simulink model "Shanthan_Heeirthan_EE469S3D_R45 (1)"  (R2023a)
settings: Solver=FixedStepDiscrete  StartTime=0.0  StopTime=120  FixedStep=dt0  RelTol=1e-3  EnableMultiTasking=on
PostLoadFcn:
  | %Set the size for the model
  | set_param(gcs,'Location',[10 10 1270 970])
  | %Set the zoom factor for the model
  | set_param(gcs,'ZoomFactor','100')
InitFcn:
  | tic
  | % Students Add call to their M-file HERE
  | Shanthan_Heeirthan_EE460_Final
  | INIT_S3D_01
StartFcn:
  | tend0=toc;
  | tic;
StopFcn:
  | tend=toc;
  | disp(['Simulation time = ' num2str(tout(end)) ' sec'])
  | disp(['Real time = ' num2str(tend) ' sec'])
  | title('DONE')
  | SCORE=round((max(0,120-tout(end)-tend0))*4+10*(40-FuelBurned)+sum(100*double(PDONE)-100*double(PDONE<.5)));
  | PlotS3D(PlotInput);
  | text(15,22,['S: ' num2str(SCORE)]);
values from neighbouring files (symbols this model uses):
  A = [0 1 0 0 0 0 ... (first row only)    [Shanthan_Heeirthan_EE460_Final (1).m]
  B = [0 0 0 ... (first row only)    [Shanthan_Heeirthan_EE460_Final (1).m]
  bm = [1 1 -1 -1 0 0 0 0; 0 0 0 0 -1 1 1 -1; -1 1 -1 1 3 -3 3 -3]    [Shanthan_Heeirthan_EE460_Final (1).m]
  C = [1 0 0 0 0 0 ... (first row only)    [Shanthan_Heeirthan_EE460_Final (1).m]
  D = [0 0 0 ... (first row only)    [Shanthan_Heeirthan_EE460_Final (1).m]
  Denchptheta = TFchptheta.Den{1}    [Shanthan_Heeirthan_EE460_Final (1).m]
  Denchpxy = TFchpxy.Den{1}    [Shanthan_Heeirthan_EE460_Final (1).m]
  Denclptheta = TFclptheta.Den{1}    [Shanthan_Heeirthan_EE460_Final (1).m]
  Denclpxy = TFclpxy.Den{1}    [Shanthan_Heeirthan_EE460_Final (1).m]
  Denlp = TFlp.Den{1}    [Shanthan_Heeirthan_EE460_Final (1).m]
  Kd = 2.1+0    (= 2.1)    [Shanthan_Heeirthan_EE460_Final (1).m]
  Ki = 0.0001    [Shanthan_Heeirthan_EE460_Final (1).m]
  Kp = 1.1+0.2    (= 1.3)    [Shanthan_Heeirthan_EE460_Final (1).m]
  L = place(A',C',ep)'    [Shanthan_Heeirthan_EE460_Final (1).m]
  Numchptheta = TFchptheta.Num{1}    [Shanthan_Heeirthan_EE460_Final (1).m]
  Numchpxy = TFchpxy.Num{1}    [Shanthan_Heeirthan_EE460_Final (1).m]
  Numclptheta = TFclptheta.Num{1}    [Shanthan_Heeirthan_EE460_Final (1).m]
  Numclpxy = TFclpxy.Num{1}    [Shanthan_Heeirthan_EE460_Final (1).m]
  Numlp = TFlp.Num{1}    [Shanthan_Heeirthan_EE460_Final (1).m]
  Pnewdata = [LVL.P1 LVL.P2 LVL.P3 LVL.P4]    [Shanthan_Heeirthan_EE460_Final (1).m]
  Sconfig = 1    [Shanthan_Heeirthan_EE460_Final (1).m]
  TFP1 = 2    [Shanthan_Heeirthan_EE460_Final (1).m]
  TFP1z = 1    [Shanthan_Heeirthan_EE460_Final (1).m]
  TFP2 = 2    [Shanthan_Heeirthan_EE460_Final (1).m]
  TFP2z = 1    [Shanthan_Heeirthan_EE460_Final (1).m]
  TFP3 = 2    [Shanthan_Heeirthan_EE460_Final (1).m]
  TFP3z = 1    [Shanthan_Heeirthan_EE460_Final (1).m]
  TFP4 = 2    [Shanthan_Heeirthan_EE460_Final (1).m]
  TFP4z = 1    [Shanthan_Heeirthan_EE460_Final (1).m]
  wcf = 2    [Shanthan_Heeirthan_EE460_Final (1).m]
  wcft = 10    [Shanthan_Heeirthan_EE460_Final (1).m]
undefined symbols (not defined in the file or in its folder): d2r, DiscIntNeverNeededParam, dt, dt0, fr, HM_S, HM_U, J, Jbase, JC0, L13, L24, LVL, M, M1, M2, M3, M4, mdti, Pdata, PTvec, r2d, SLIM, SQ, SSF, TOLdata, ULIM
libraries: simulink x85, aerolibanimutils x1, matrix_library x1
(part 5 of 7)

== system Shanthan_Heeirthan_EE469S3D_R45 (1)/S3D_Plant/Sensors/CASE1/Xaccel/CURRENT ==
  In1 : Inport
  Action Port : ActionPort  ActionPortLabel=else
  Out1 : Outport
  wires:
  In1/1 -> Out1/1

== system Shanthan_Heeirthan_EE469S3D_R45 (1)/S3D_Plant/Sensors/CASE1/Xaccel/MAX ==
  Action Port : ActionPort  ActionPortLabel=elseif(u1 > 0.5 & u1 < 1.5)
  Constant : Constant  Value=SLIM(3,2)  SampleTime=dt0
  Out1 : Outport
  wires:
  Constant/1 -> Out1/1

== system Shanthan_Heeirthan_EE469S3D_R45 (1)/S3D_Plant/Sensors/CASE1/Xaccel/MIN ==
  Action Port : ActionPort  ActionPortLabel=if(u1 < -0.5)
  Constant : Constant  Value=SLIM(3,1)  SampleTime=dt0
  Out1 : Outport
  wires:
  Constant/1 -> Out1/1

== system Shanthan_Heeirthan_EE469S3D_R45 (1)/S3D_Plant/Sensors/CASE1/Xpos1/CURRENT ==
  In1 : Inport
  Action Port : ActionPort  ActionPortLabel=else
  Out1 : Outport
  wires:
  In1/1 -> Out1/1

== system Shanthan_Heeirthan_EE469S3D_R45 (1)/S3D_Plant/Sensors/CASE1/Xpos1/MAX ==
  Action Port : ActionPort  ActionPortLabel=elseif(u1 > 0.5 & u1 < 1.5)
  Constant : Constant  Value=SLIM(1,2)  SampleTime=dt0
  Out1 : Outport
  wires:
  Constant/1 -> Out1/1

== system Shanthan_Heeirthan_EE469S3D_R45 (1)/S3D_Plant/Sensors/CASE1/Xpos1/MIN ==
  Action Port : ActionPort  ActionPortLabel=if(u1 < -0.5)
  Constant : Constant  Value=SLIM(1,1)  SampleTime=dt0
  Out1 : Outport
  wires:
  Constant/1 -> Out1/1

== system Shanthan_Heeirthan_EE469S3D_R45 (1)/S3D_Plant/Sensors/CASE1/Xvel/CURRENT ==
  In1 : Inport
  Action Port : ActionPort  ActionPortLabel=else
  Out1 : Outport
  wires:
  In1/1 -> Out1/1

== system Shanthan_Heeirthan_EE469S3D_R45 (1)/S3D_Plant/Sensors/CASE1/Xvel/MAX ==
  Action Port : ActionPort  ActionPortLabel=elseif(u1 > 0.5 & u1 < 1.5)
  Constant : Constant  Value=SLIM(2,2)  SampleTime=dt0
  Out1 : Outport
  wires:
  Constant/1 -> Out1/1

== system Shanthan_Heeirthan_EE469S3D_R45 (1)/S3D_Plant/Sensors/CASE1/Xvel/MIN ==
  Action Port : ActionPort  ActionPortLabel=if(u1 < -0.5)
  Constant : Constant  Value=SLIM(2,1)  SampleTime=dt0
  Out1 : Outport
  wires:
  Constant/1 -> Out1/1

== system Shanthan_Heeirthan_EE469S3D_R45 (1)/S3D_Plant/Sensors/CASE1/Yaccel/CURRENT ==
  In1 : Inport
  Action Port : ActionPort  ActionPortLabel=else
  Out1 : Outport
  wires:
  In1/1 -> Out1/1

== system Shanthan_Heeirthan_EE469S3D_R45 (1)/S3D_Plant/Sensors/CASE1/Yaccel/MAX ==
  Action Port : ActionPort  ActionPortLabel=elseif(u1 > 0.5 & u1 < 1.5)
  Constant : Constant  Value=SLIM(6,2)  SampleTime=dt0
  Out1 : Outport
  wires:
  Constant/1 -> Out1/1

== system Shanthan_Heeirthan_EE469S3D_R45 (1)/S3D_Plant/Sensors/CASE1/Yaccel/MIN ==
  Action Port : ActionPort  ActionPortLabel=if(u1 < -0.5)
  Constant : Constant  Value=SLIM(6,1)  SampleTime=dt0
  Out1 : Outport
  wires:
  Constant/1 -> Out1/1

== system Shanthan_Heeirthan_EE469S3D_R45 (1)/S3D_Plant/Sensors/CASE1/Ypos1/CURRENT ==
  In1 : Inport
  Action Port : ActionPort  ActionPortLabel=else
  Out1 : Outport
  wires:
  In1/1 -> Out1/1

== system Shanthan_Heeirthan_EE469S3D_R45 (1)/S3D_Plant/Sensors/CASE1/Ypos1/MAX ==
  Action Port : ActionPort  ActionPortLabel=elseif(u1 > 0.5 & u1 < 1.5)
  Constant : Constant  Value=SLIM(4,2)  SampleTime=dt0
  Out1 : Outport
  wires:
  Constant/1 -> Out1/1

== system Shanthan_Heeirthan_EE469S3D_R45 (1)/S3D_Plant/Sensors/CASE1/Ypos1/MIN ==
  Action Port : ActionPort  ActionPortLabel=if(u1 < -0.5)
  Constant : Constant  Value=SLIM(4,1)  SampleTime=dt0
  Out1 : Outport
  wires:
  Constant/1 -> Out1/1

== system Shanthan_Heeirthan_EE469S3D_R45 (1)/S3D_Plant/Sensors/CASE1/Yvel/CURRENT ==
  In1 : Inport
  Action Port : ActionPort  ActionPortLabel=else
  Out1 : Outport
  wires:
  In1/1 -> Out1/1

== system Shanthan_Heeirthan_EE469S3D_R45 (1)/S3D_Plant/Sensors/CASE1/Yvel/MAX ==
  Action Port : ActionPort  ActionPortLabel=elseif(u1 > 0.5 & u1 < 1.5)
  Constant : Constant  Value=SLIM(5,2)  SampleTime=dt0
  Out1 : Outport
  wires:
  Constant/1 -> Out1/1

== system Shanthan_Heeirthan_EE469S3D_R45 (1)/S3D_Plant/Sensors/CASE1/Yvel/MIN ==
  Action Port : ActionPort  ActionPortLabel=if(u1 < -0.5)
  Constant : Constant  Value=SLIM(5,1)  SampleTime=dt0
  Out1 : Outport
  wires:
  Constant/1 -> Out1/1

== system Shanthan_Heeirthan_EE469S3D_R45 (1)/S3D_Plant/Sensors/CASE2/THTpos1/CURRENT ==
  In1 : Inport
  Action Port : ActionPort  ActionPortLabel=else
  Out1 : Outport
  wires:
  In1/1 -> Out1/1

== system Shanthan_Heeirthan_EE469S3D_R45 (1)/S3D_Plant/Sensors/CASE2/THTpos1/MAX ==
  Action Port : ActionPort  ActionPortLabel=elseif(u1 > 0.5 & u1 < 1.5)
  Constant : Constant  Value=SLIM(7,2)  SampleTime=dt0
  Out1 : Outport
  wires:
  Constant/1 -> Out1/1

== system Shanthan_Heeirthan_EE469S3D_R45 (1)/S3D_Plant/Sensors/CASE2/THTpos1/MIN ==
  Action Port : ActionPort  ActionPortLabel=if(u1 < -0.5)
  Constant : Constant  Value=SLIM(7,1)  SampleTime=dt0
  Out1 : Outport
  wires:
  Constant/1 -> Out1/1

== system Shanthan_Heeirthan_EE469S3D_R45 (1)/S3D_Plant/Sensors/CASE2/THTpos2/CURRENT ==
  In1 : Inport
  Action Port : ActionPort  ActionPortLabel=else
  Out1 : Outport
  wires:
  In1/1 -> Out1/1

== system Shanthan_Heeirthan_EE469S3D_R45 (1)/S3D_Plant/Sensors/CASE2/THTpos2/MAX ==
  Action Port : ActionPort  ActionPortLabel=elseif(u1 > 0.5 & u1 < 1.5)
  Constant : Constant  Value=SLIM(7,2)  SampleTime=dt0
  Out1 : Outport
  wires:
  Constant/1 -> Out1/1

== system Shanthan_Heeirthan_EE469S3D_R45 (1)/S3D_Plant/Sensors/CASE2/THTpos2/MIN ==
  Action Port : ActionPort  ActionPortLabel=if(u1 < -0.5)
  Constant : Constant  Value=SLIM(7,1)  SampleTime=dt0
  Out1 : Outport
  wires:
  Constant/1 -> Out1/1

== system Shanthan_Heeirthan_EE469S3D_R45 (1)/S3D_Plant/Sensors/CASE2/THTvel/CURRENT ==
  In1 : Inport
  Action Port : ActionPort  ActionPortLabel=else
  Out1 : Outport
  wires:
  In1/1 -> Out1/1

== system Shanthan_Heeirthan_EE469S3D_R45 (1)/S3D_Plant/Sensors/CASE2/THTvel/MAX ==
  Action Port : ActionPort  ActionPortLabel=elseif(u1 > 0.5 & u1 < 1.5)
  Constant : Constant  Value=SLIM(8,2)  SampleTime=dt0
  Out1 : Outport
  wires:
  Constant/1 -> Out1/1

== system Shanthan_Heeirthan_EE469S3D_R45 (1)/S3D_Plant/Sensors/CASE2/THTvel/MIN ==
  Action Port : ActionPort  ActionPortLabel=if(u1 < -0.5)
  Constant : Constant  Value=SLIM(8,1)  SampleTime=dt0
  Out1 : Outport
  wires:
  Constant/1 -> Out1/1

== system Shanthan_Heeirthan_EE469S3D_R45 (1)/S3D_Plant/Sensors/CASE2/Xpos1/CURRENT ==
  In1 : Inport
  Action Port : ActionPort  ActionPortLabel=else
  Out1 : Outport
  wires:
  In1/1 -> Out1/1

== system Shanthan_Heeirthan_EE469S3D_R45 (1)/S3D_Plant/Sensors/CASE2/Xpos1/MAX ==
  Action Port : ActionPort  ActionPortLabel=elseif(u1 > 0.5 & u1 < 1.5)
  Constant : Constant  Value=SLIM(1,2)  SampleTime=dt0
  Out1 : Outport
  wires:
  Constant/1 -> Out1/1

== system Shanthan_Heeirthan_EE469S3D_R45 (1)/S3D_Plant/Sensors/CASE2/Xpos1/MIN ==
  Action Port : ActionPort  ActionPortLabel=if(u1 < -0.5)
  Constant : Constant  Value=SLIM(1,1)  SampleTime=dt0
  Out1 : Outport
  wires:
  Constant/1 -> Out1/1

== system Shanthan_Heeirthan_EE469S3D_R45 (1)/S3D_Plant/Sensors/CASE2/Xpos2/CURRENT ==
  In1 : Inport
  Action Port : ActionPort  ActionPortLabel=else
  Out1 : Outport
  wires:
  In1/1 -> Out1/1

== system Shanthan_Heeirthan_EE469S3D_R45 (1)/S3D_Plant/Sensors/CASE2/Xpos2/MAX ==
  Action Port : ActionPort  ActionPortLabel=elseif(u1 > 0.5 & u1 < 1.5)
  Constant : Constant  Value=SLIM(1,2)  SampleTime=dt0
  Out1 : Outport
  wires:
  Constant/1 -> Out1/1

== system Shanthan_Heeirthan_EE469S3D_R45 (1)/S3D_Plant/Sensors/CASE2/Xpos2/MIN ==
  Action Port : ActionPort  ActionPortLabel=if(u1 < -0.5)
  Constant : Constant  Value=SLIM(1,1)  SampleTime=dt0
  Out1 : Outport
  wires:
  Constant/1 -> Out1/1

== system Shanthan_Heeirthan_EE469S3D_R45 (1)/S3D_Plant/Sensors/CASE2/Xvel/CURRENT ==
  In1 : Inport
  Action Port : ActionPort  ActionPortLabel=else
  Out1 : Outport
  wires:
  In1/1 -> Out1/1

== system Shanthan_Heeirthan_EE469S3D_R45 (1)/S3D_Plant/Sensors/CASE2/Xvel/MAX ==
  Action Port : ActionPort  ActionPortLabel=elseif(u1 > 0.5 & u1 < 1.5)
  Constant : Constant  Value=SLIM(2,2)  SampleTime=dt0
  Out1 : Outport
  wires:
  Constant/1 -> Out1/1

== system Shanthan_Heeirthan_EE469S3D_R45 (1)/S3D_Plant/Sensors/CASE2/Xvel/MIN ==
  Action Port : ActionPort  ActionPortLabel=if(u1 < -0.5)
  Constant : Constant  Value=SLIM(2,1)  SampleTime=dt0
  Out1 : Outport
  wires:
  Constant/1 -> Out1/1

== system Shanthan_Heeirthan_EE469S3D_R45 (1)/S3D_Plant/Sensors/CASE2/Ypos1/CURRENT ==
  In1 : Inport
  Action Port : ActionPort  ActionPortLabel=else
  Out1 : Outport
  wires:
  In1/1 -> Out1/1

== system Shanthan_Heeirthan_EE469S3D_R45 (1)/S3D_Plant/Sensors/CASE2/Ypos1/MAX ==
  Action Port : ActionPort  ActionPortLabel=elseif(u1 > 0.5 & u1 < 1.5)
  Constant : Constant  Value=SLIM(4,2)  SampleTime=dt0
  Out1 : Outport
  wires:
  Constant/1 -> Out1/1

== system Shanthan_Heeirthan_EE469S3D_R45 (1)/S3D_Plant/Sensors/CASE2/Ypos1/MIN ==
  Action Port : ActionPort  ActionPortLabel=if(u1 < -0.5)
  Constant : Constant  Value=SLIM(4,1)  SampleTime=dt0
  Out1 : Outport
  wires:
  Constant/1 -> Out1/1

== system Shanthan_Heeirthan_EE469S3D_R45 (1)/S3D_Plant/Sensors/CASE2/Ypos2/CURRENT ==
  In1 : Inport
  Action Port : ActionPort  ActionPortLabel=else
  Out1 : Outport
  wires:
  In1/1 -> Out1/1

== system Shanthan_Heeirthan_EE469S3D_R45 (1)/S3D_Plant/Sensors/CASE2/Ypos2/MAX ==
  Action Port : ActionPort  ActionPortLabel=elseif(u1 > 0.5 & u1 < 1.5)
  Constant : Constant  Value=SLIM(4,2)  SampleTime=dt0
  Out1 : Outport
  wires:
  Constant/1 -> Out1/1

== system Shanthan_Heeirthan_EE469S3D_R45 (1)/S3D_Plant/Sensors/CASE2/Ypos2/MIN ==
  Action Port : ActionPort  ActionPortLabel=if(u1 < -0.5)
  Constant : Constant  Value=SLIM(4,1)  SampleTime=dt0
  Out1 : Outport
  wires:
  Constant/1 -> Out1/1

== system Shanthan_Heeirthan_EE469S3D_R45 (1)/S3D_Plant/Sensors/CASE2/Yvel/CURRENT ==
  In1 : Inport
  Action Port : ActionPort  ActionPortLabel=else
  Out1 : Outport
  wires:
  In1/1 -> Out1/1

== system Shanthan_Heeirthan_EE469S3D_R45 (1)/S3D_Plant/Sensors/CASE2/Yvel/MAX ==
  Action Port : ActionPort  ActionPortLabel=elseif(u1 > 0.5 & u1 < 1.5)
  Constant : Constant  Value=SLIM(5,2)  SampleTime=dt0
  Out1 : Outport
  wires:
  Constant/1 -> Out1/1

== system Shanthan_Heeirthan_EE469S3D_R45 (1)/S3D_Plant/Sensors/CASE2/Yvel/MIN ==
  Action Port : ActionPort  ActionPortLabel=if(u1 < -0.5)
  Constant : Constant  Value=SLIM(5,1)  SampleTime=dt0
  Out1 : Outport
  wires:
  Constant/1 -> Out1/1

== system Shanthan_Heeirthan_EE469S3D_R45 (1)/S3D_Plant/Sensors/CASE3/THTpos1/CURRENT ==
  In1 : Inport
  Action Port : ActionPort  ActionPortLabel=else
  Out1 : Outport
  wires:
  In1/1 -> Out1/1

== system Shanthan_Heeirthan_EE469S3D_R45 (1)/S3D_Plant/Sensors/CASE3/THTpos1/MAX ==
  Action Port : ActionPort  ActionPortLabel=elseif(u1 > 0.5 & u1 < 1.5)
  Constant : Constant  Value=SLIM(7,2)  SampleTime=dt0
  Out1 : Outport
  wires:
  Constant/1 -> Out1/1

== system Shanthan_Heeirthan_EE469S3D_R45 (1)/S3D_Plant/Sensors/CASE3/THTpos1/MIN ==
  Action Port : ActionPort  ActionPortLabel=if(u1 < -0.5)
  Constant : Constant  Value=SLIM(7,1)  SampleTime=dt0
  Out1 : Outport
  wires:
  Constant/1 -> Out1/1

== system Shanthan_Heeirthan_EE469S3D_R45 (1)/S3D_Plant/Sensors/CASE3/THTpos2/CURRENT ==
  In1 : Inport
  Action Port : ActionPort  ActionPortLabel=else
  Out1 : Outport
  wires:
  In1/1 -> Out1/1

== system Shanthan_Heeirthan_EE469S3D_R45 (1)/S3D_Plant/Sensors/CASE3/THTpos2/MAX ==
  Action Port : ActionPort  ActionPortLabel=elseif(u1 > 0.5 & u1 < 1.5)
  Constant : Constant  Value=SLIM(7,2)  SampleTime=dt0
  Out1 : Outport
  wires:
  Constant/1 -> Out1/1

== system Shanthan_Heeirthan_EE469S3D_R45 (1)/S3D_Plant/Sensors/CASE3/THTpos2/MIN ==
  Action Port : ActionPort  ActionPortLabel=if(u1 < -0.5)
  Constant : Constant  Value=SLIM(7,1)  SampleTime=dt0
  Out1 : Outport
  wires:
  Constant/1 -> Out1/1

== system Shanthan_Heeirthan_EE469S3D_R45 (1)/S3D_Plant/Sensors/CASE3/THTpos3/CURRENT ==
  In1 : Inport
  Action Port : ActionPort  ActionPortLabel=else
  Out1 : Outport
  wires:
  In1/1 -> Out1/1

== system Shanthan_Heeirthan_EE469S3D_R45 (1)/S3D_Plant/Sensors/CASE3/THTpos3/MAX ==
  Action Port : ActionPort  ActionPortLabel=elseif(u1 > 0.5 & u1 < 1.5)
  Constant : Constant  Value=SLIM(7,2)  SampleTime=dt0
  Out1 : Outport
  wires:
  Constant/1 -> Out1/1

== system Shanthan_Heeirthan_EE469S3D_R45 (1)/S3D_Plant/Sensors/CASE3/THTpos3/MIN ==
  Action Port : ActionPort  ActionPortLabel=if(u1 < -0.5)
  Constant : Constant  Value=SLIM(7,1)  SampleTime=dt0
  Out1 : Outport
  wires:
  Constant/1 -> Out1/1

== system Shanthan_Heeirthan_EE469S3D_R45 (1)/S3D_Plant/Sensors/CASE3/Xpos1/CURRENT ==
  In1 : Inport
  Action Port : ActionPort  ActionPortLabel=else
  Out1 : Outport
  wires:
  In1/1 -> Out1/1

== system Shanthan_Heeirthan_EE469S3D_R45 (1)/S3D_Plant/Sensors/CASE3/Xpos1/MAX ==
  Action Port : ActionPort  ActionPortLabel=elseif(u1 > 0.5 & u1 < 1.5)
  Constant : Constant  Value=SLIM(1,2)  SampleTime=dt0
  Out1 : Outport
  wires:
  Constant/1 -> Out1/1

== system Shanthan_Heeirthan_EE469S3D_R45 (1)/S3D_Plant/Sensors/CASE3/Xpos1/MIN ==
  Action Port : ActionPort  ActionPortLabel=if(u1 < -0.5)
  Constant : Constant  Value=SLIM(1,1)  SampleTime=dt0
  Out1 : Outport
  wires:
  Constant/1 -> Out1/1

== system Shanthan_Heeirthan_EE469S3D_R45 (1)/S3D_Plant/Sensors/CASE3/Xpos2/CURRENT ==
  In1 : Inport
  Action Port : ActionPort  ActionPortLabel=else
  Out1 : Outport
  wires:
  In1/1 -> Out1/1

== system Shanthan_Heeirthan_EE469S3D_R45 (1)/S3D_Plant/Sensors/CASE3/Xpos2/MAX ==
  Action Port : ActionPort  ActionPortLabel=elseif(u1 > 0.5 & u1 < 1.5)
  Constant : Constant  Value=SLIM(1,2)  SampleTime=dt0
  Out1 : Outport
  wires:
  Constant/1 -> Out1/1

== system Shanthan_Heeirthan_EE469S3D_R45 (1)/S3D_Plant/Sensors/CASE3/Xpos2/MIN ==
  Action Port : ActionPort  ActionPortLabel=if(u1 < -0.5)
  Constant : Constant  Value=SLIM(1,1)  SampleTime=dt0
  Out1 : Outport
  wires:
  Constant/1 -> Out1/1

== system Shanthan_Heeirthan_EE469S3D_R45 (1)/S3D_Plant/Sensors/CASE3/Xpos3/CURRENT ==
  In1 : Inport
  Action Port : ActionPort  ActionPortLabel=else
  Out1 : Outport
  wires:
  In1/1 -> Out1/1

== system Shanthan_Heeirthan_EE469S3D_R45 (1)/S3D_Plant/Sensors/CASE3/Xpos3/MAX ==
  Action Port : ActionPort  ActionPortLabel=elseif(u1 > 0.5 & u1 < 1.5)
  Constant : Constant  Value=SLIM(1,2)  SampleTime=dt0
  Out1 : Outport
  wires:
  Constant/1 -> Out1/1

== system Shanthan_Heeirthan_EE469S3D_R45 (1)/S3D_Plant/Sensors/CASE3/Xpos3/MIN ==
  Action Port : ActionPort  ActionPortLabel=if(u1 < -0.5)
  Constant : Constant  Value=SLIM(1,1)  SampleTime=dt0
  Out1 : Outport
  wires:
  Constant/1 -> Out1/1

== system Shanthan_Heeirthan_EE469S3D_R45 (1)/S3D_Plant/Sensors/CASE3/Ypos1/CURRENT ==
  In1 : Inport
  Action Port : ActionPort  ActionPortLabel=else
  Out1 : Outport
  wires:
  In1/1 -> Out1/1

== system Shanthan_Heeirthan_EE469S3D_R45 (1)/S3D_Plant/Sensors/CASE3/Ypos1/MAX ==
  Action Port : ActionPort  ActionPortLabel=elseif(u1 > 0.5 & u1 < 1.5)
  Constant : Constant  Value=SLIM(4,2)  SampleTime=dt0
  Out1 : Outport
  wires:
  Constant/1 -> Out1/1

== system Shanthan_Heeirthan_EE469S3D_R45 (1)/S3D_Plant/Sensors/CASE3/Ypos1/MIN ==
  Action Port : ActionPort  ActionPortLabel=if(u1 < -0.5)
  Constant : Constant  Value=SLIM(4,1)  SampleTime=dt0
  Out1 : Outport
  wires:
  Constant/1 -> Out1/1

== system Shanthan_Heeirthan_EE469S3D_R45 (1)/S3D_Plant/Sensors/CASE3/Ypos2/CURRENT ==
  In1 : Inport
  Action Port : ActionPort  ActionPortLabel=else
  Out1 : Outport
  wires:
  In1/1 -> Out1/1

== system Shanthan_Heeirthan_EE469S3D_R45 (1)/S3D_Plant/Sensors/CASE3/Ypos2/MAX ==
  Action Port : ActionPort  ActionPortLabel=elseif(u1 > 0.5 & u1 < 1.5)
  Constant : Constant  Value=SLIM(4,2)  SampleTime=dt0
  Out1 : Outport
  wires:
  Constant/1 -> Out1/1

== system Shanthan_Heeirthan_EE469S3D_R45 (1)/S3D_Plant/Sensors/CASE3/Ypos2/MIN ==
  Action Port : ActionPort  ActionPortLabel=if(u1 < -0.5)
  Constant : Constant  Value=SLIM(4,1)  SampleTime=dt0
  Out1 : Outport
  wires:
  Constant/1 -> Out1/1

== system Shanthan_Heeirthan_EE469S3D_R45 (1)/S3D_Plant/Sensors/CASE3/Ypos3/CURRENT ==
  In1 : Inport
  Action Port : ActionPort  ActionPortLabel=else
  Out1 : Outport
  wires:
  In1/1 -> Out1/1

== system Shanthan_Heeirthan_EE469S3D_R45 (1)/S3D_Plant/Sensors/CASE3/Ypos3/MAX ==
  Action Port : ActionPort  ActionPortLabel=elseif(u1 > 0.5 & u1 < 1.5)
  Constant : Constant  Value=SLIM(4,2)  SampleTime=dt0
  Out1 : Outport
  wires:
  Constant/1 -> Out1/1

== system Shanthan_Heeirthan_EE469S3D_R45 (1)/S3D_Plant/Sensors/CASE3/Ypos3/MIN ==
  Action Port : ActionPort  ActionPortLabel=if(u1 < -0.5)
  Constant : Constant  Value=SLIM(4,1)  SampleTime=dt0
  Out1 : Outport
  wires:
  Constant/1 -> Out1/1

== system Shanthan_Heeirthan_EE469S3D_R45 (1)/S3D_Plant/ThrusterValues/FailModes/Ufail1/CURRENT ==
  In1 : Inport
  Action Port : ActionPort  ActionPortLabel=else
  Out1 : Outport
  wires:
  In1/1 -> Out1/1

== system Shanthan_Heeirthan_EE469S3D_R45 (1)/S3D_Plant/ThrusterValues/FailModes/Ufail1/FailLogic ==
  BeforeFail : Inport
  FuelRemaining : Inport  Port=2
  FailMode : Inport  Port=3
  Abs : Abs  SaturateOnIntegerOverflow=off
  Compare To Constant : simulink/Logic and Bit Operations/Compare To Constant  relop=<=  const=0.5  OutDataTypeStr=boolean
  Logical Operator : Logic  Operator=OR  AllPortsSameDT=off  OutDataTypeStr=boolean
  Logical Operator1 : Logic  AllPortsSameDT=off  OutDataTypeStr=boolean
  NoFail : Outport
  wires:
  FailMode/1 -> Abs/1
  Logical Operator1/1 -> NoFail/1
  Compare To Constant/1 -> Logical Operator/2
  BeforeFail/1 -> Logical Operator/1
  Abs/1 -> Compare To Constant/1
  Logical Operator/1 -> Logical Operator1/1
  FuelRemaining/1 -> Logical Operator1/2

== system Shanthan_Heeirthan_EE469S3D_R45 (1)/S3D_Plant/ThrusterValues/FailModes/Ufail1/MAX ==
  Action Port : ActionPort  ActionPortLabel=elseif(u1 > 0.5 & u1 < 1.5)
  Constant : Constant  Value=ULIM(Udx,2)  SampleTime=dt0
  Out1 : Outport
  wires:
  Constant/1 -> Out1/1

== system Shanthan_Heeirthan_EE469S3D_R45 (1)/S3D_Plant/ThrusterValues/FailModes/Ufail1/MIN ==
  Action Port : ActionPort  ActionPortLabel=if(u1 < -0.5)
  Constant : Constant  Value=ULIM(Udx,1)  SampleTime=dt0
  Out1 : Outport
  wires:
  Constant/1 -> Out1/1

== system Shanthan_Heeirthan_EE469S3D_R45 (1)/S3D_Plant/ThrusterValues/FailModes/Ufail10/CURRENT ==
  In1 : Inport
  Action Port : ActionPort  ActionPortLabel=else
  Out1 : Outport
  wires:
  In1/1 -> Out1/1

== system Shanthan_Heeirthan_EE469S3D_R45 (1)/S3D_Plant/ThrusterValues/FailModes/Ufail10/FailLogic ==
  BeforeFail : Inport
  FuelRemaining : Inport  Port=2
  FailMode : Inport  Port=3
  Abs : Abs  SaturateOnIntegerOverflow=off
  Compare To Constant : simulink/Logic and Bit Operations/Compare To Constant  relop=<=  const=0.5  OutDataTypeStr=boolean
  Logical Operator : Logic  Operator=OR  AllPortsSameDT=off  OutDataTypeStr=boolean
  Logical Operator1 : Logic  AllPortsSameDT=off  OutDataTypeStr=boolean
  NoFail : Outport
  wires:
  FailMode/1 -> Abs/1
  Logical Operator1/1 -> NoFail/1
  Compare To Constant/1 -> Logical Operator/2
  BeforeFail/1 -> Logical Operator/1
  Abs/1 -> Compare To Constant/1
  Logical Operator/1 -> Logical Operator1/1
  FuelRemaining/1 -> Logical Operator1/2

== system Shanthan_Heeirthan_EE469S3D_R45 (1)/S3D_Plant/ThrusterValues/FailModes/Ufail10/MAX ==
  Action Port : ActionPort  ActionPortLabel=elseif(u1 > 0.5 & u1 < 1.5)
  Constant : Constant  Value=ULIM(Udx,2)  SampleTime=dt0
  Out1 : Outport
  wires:
  Constant/1 -> Out1/1

== system Shanthan_Heeirthan_EE469S3D_R45 (1)/S3D_Plant/ThrusterValues/FailModes/Ufail10/MIN ==
  Action Port : ActionPort  ActionPortLabel=if(u1 < -0.5)
  Constant : Constant  Value=ULIM(Udx,1)  SampleTime=dt0
  Out1 : Outport
  wires:
  Constant/1 -> Out1/1

== system Shanthan_Heeirthan_EE469S3D_R45 (1)/S3D_Plant/ThrusterValues/FailModes/Ufail2/CURRENT ==
  In1 : Inport
  Action Port : ActionPort  ActionPortLabel=else
  Out1 : Outport
  wires:
  In1/1 -> Out1/1

== system Shanthan_Heeirthan_EE469S3D_R45 (1)/S3D_Plant/ThrusterValues/FailModes/Ufail2/FailLogic ==
  BeforeFail : Inport
  FuelRemaining : Inport  Port=2
  FailMode : Inport  Port=3
  Abs : Abs  SaturateOnIntegerOverflow=off
  Compare To Constant : simulink/Logic and Bit Operations/Compare To Constant  relop=<=  const=0.5  OutDataTypeStr=boolean
  Logical Operator : Logic  Operator=OR  AllPortsSameDT=off  OutDataTypeStr=boolean
  Logical Operator1 : Logic  AllPortsSameDT=off  OutDataTypeStr=boolean
  NoFail : Outport
  wires:
  FailMode/1 -> Abs/1
  Logical Operator1/1 -> NoFail/1
  Compare To Constant/1 -> Logical Operator/2
  BeforeFail/1 -> Logical Operator/1
  Abs/1 -> Compare To Constant/1
  Logical Operator/1 -> Logical Operator1/1
  FuelRemaining/1 -> Logical Operator1/2

== system Shanthan_Heeirthan_EE469S3D_R45 (1)/S3D_Plant/ThrusterValues/FailModes/Ufail2/MAX ==
  Action Port : ActionPort  ActionPortLabel=elseif(u1 > 0.5 & u1 < 1.5)
  Constant : Constant  Value=ULIM(Udx,2)  SampleTime=dt0
  Out1 : Outport
  wires:
  Constant/1 -> Out1/1

== system Shanthan_Heeirthan_EE469S3D_R45 (1)/S3D_Plant/ThrusterValues/FailModes/Ufail2/MIN ==
  Action Port : ActionPort  ActionPortLabel=if(u1 < -0.5)
  Constant : Constant  Value=ULIM(Udx,1)  SampleTime=dt0
  Out1 : Outport
  wires:
  Constant/1 -> Out1/1

== system Shanthan_Heeirthan_EE469S3D_R45 (1)/S3D_Plant/ThrusterValues/FailModes/Ufail3/CURRENT ==
  In1 : Inport
  Action Port : ActionPort  ActionPortLabel=else
  Out1 : Outport
  wires:
  In1/1 -> Out1/1

== system Shanthan_Heeirthan_EE469S3D_R45 (1)/S3D_Plant/ThrusterValues/FailModes/Ufail3/FailLogic ==
  BeforeFail : Inport
  FuelRemaining : Inport  Port=2
  FailMode : Inport  Port=3
  Abs : Abs  SaturateOnIntegerOverflow=off
  Compare To Constant : simulink/Logic and Bit Operations/Compare To Constant  relop=<=  const=0.5  OutDataTypeStr=boolean
  Logical Operator : Logic  Operator=OR  AllPortsSameDT=off  OutDataTypeStr=boolean
  Logical Operator1 : Logic  AllPortsSameDT=off  OutDataTypeStr=boolean
  NoFail : Outport
  wires:
  FailMode/1 -> Abs/1
  Logical Operator1/1 -> NoFail/1
  Compare To Constant/1 -> Logical Operator/2
  BeforeFail/1 -> Logical Operator/1
  Abs/1 -> Compare To Constant/1
  Logical Operator/1 -> Logical Operator1/1
  FuelRemaining/1 -> Logical Operator1/2

== system Shanthan_Heeirthan_EE469S3D_R45 (1)/S3D_Plant/ThrusterValues/FailModes/Ufail3/MAX ==
  Action Port : ActionPort  ActionPortLabel=elseif(u1 > 0.5 & u1 < 1.5)
  Constant : Constant  Value=ULIM(Udx,2)  SampleTime=dt0
  Out1 : Outport
  wires:
  Constant/1 -> Out1/1

== system Shanthan_Heeirthan_EE469S3D_R45 (1)/S3D_Plant/ThrusterValues/FailModes/Ufail3/MIN ==
  Action Port : ActionPort  ActionPortLabel=if(u1 < -0.5)
  Constant : Constant  Value=ULIM(Udx,1)  SampleTime=dt0
  Out1 : Outport
  wires:
  Constant/1 -> Out1/1

== system Shanthan_Heeirthan_EE469S3D_R45 (1)/S3D_Plant/ThrusterValues/FailModes/Ufail4/CURRENT ==
  In1 : Inport
  Action Port : ActionPort  ActionPortLabel=else
  Out1 : Outport
  wires:
  In1/1 -> Out1/1

== system Shanthan_Heeirthan_EE469S3D_R45 (1)/S3D_Plant/ThrusterValues/FailModes/Ufail4/FailLogic ==
  BeforeFail : Inport
  FuelRemaining : Inport  Port=2
  FailMode : Inport  Port=3
  Abs : Abs  SaturateOnIntegerOverflow=off
  Compare To Constant : simulink/Logic and Bit Operations/Compare To Constant  relop=<=  const=0.5  OutDataTypeStr=boolean
  Logical Operator : Logic  Operator=OR  AllPortsSameDT=off  OutDataTypeStr=boolean
  Logical Operator1 : Logic  AllPortsSameDT=off  OutDataTypeStr=boolean
  NoFail : Outport
  wires:
  FailMode/1 -> Abs/1
  Logical Operator1/1 -> NoFail/1
  Compare To Constant/1 -> Logical Operator/2
  BeforeFail/1 -> Logical Operator/1
  Abs/1 -> Compare To Constant/1
  Logical Operator/1 -> Logical Operator1/1
  FuelRemaining/1 -> Logical Operator1/2

== system Shanthan_Heeirthan_EE469S3D_R45 (1)/S3D_Plant/ThrusterValues/FailModes/Ufail4/MAX ==
  Action Port : ActionPort  ActionPortLabel=elseif(u1 > 0.5 & u1 < 1.5)
  Constant : Constant  Value=ULIM(Udx,2)  SampleTime=dt0
  Out1 : Outport
  wires:
  Constant/1 -> Out1/1

== system Shanthan_Heeirthan_EE469S3D_R45 (1)/S3D_Plant/ThrusterValues/FailModes/Ufail4/MIN ==
  Action Port : ActionPort  ActionPortLabel=if(u1 < -0.5)
  Constant : Constant  Value=ULIM(Udx,1)  SampleTime=dt0
  Out1 : Outport
  wires:
  Constant/1 -> Out1/1

== system Shanthan_Heeirthan_EE469S3D_R45 (1)/S3D_Plant/ThrusterValues/FailModes/Ufail5/CURRENT ==
  In1 : Inport
  Action Port : ActionPort  ActionPortLabel=else
  Out1 : Outport
  wires:
  In1/1 -> Out1/1

== system Shanthan_Heeirthan_EE469S3D_R45 (1)/S3D_Plant/ThrusterValues/FailModes/Ufail5/FailLogic ==
  BeforeFail : Inport
  FuelRemaining : Inport  Port=2
  FailMode : Inport  Port=3
  Abs : Abs  SaturateOnIntegerOverflow=off
  Compare To Constant : simulink/Logic and Bit Operations/Compare To Constant  relop=<=  const=0.5  OutDataTypeStr=boolean
  Logical Operator : Logic  Operator=OR  AllPortsSameDT=off  OutDataTypeStr=boolean
  Logical Operator1 : Logic  AllPortsSameDT=off  OutDataTypeStr=boolean
  NoFail : Outport
  wires:
  FailMode/1 -> Abs/1
  Logical Operator1/1 -> NoFail/1
  Compare To Constant/1 -> Logical Operator/2
  BeforeFail/1 -> Logical Operator/1
  Abs/1 -> Compare To Constant/1
  Logical Operator/1 -> Logical Operator1/1
  FuelRemaining/1 -> Logical Operator1/2

== system Shanthan_Heeirthan_EE469S3D_R45 (1)/S3D_Plant/ThrusterValues/FailModes/Ufail5/MAX ==
  Action Port : ActionPort  ActionPortLabel=elseif(u1 > 0.5 & u1 < 1.5)
  Constant : Constant  Value=ULIM(Udx,2)  SampleTime=dt0
  Out1 : Outport
  wires:
  Constant/1 -> Out1/1

== system Shanthan_Heeirthan_EE469S3D_R45 (1)/S3D_Plant/ThrusterValues/FailModes/Ufail5/MIN ==
  Action Port : ActionPort  ActionPortLabel=if(u1 < -0.5)
  Constant : Constant  Value=ULIM(Udx,1)  SampleTime=dt0
  Out1 : Outport
  wires:
  Constant/1 -> Out1/1

== system Shanthan_Heeirthan_EE469S3D_R45 (1)/S3D_Plant/ThrusterValues/FailModes/Ufail6/CURRENT ==
  In1 : Inport
  Action Port : ActionPort  ActionPortLabel=else
  Out1 : Outport
  wires:
  In1/1 -> Out1/1

== system Shanthan_Heeirthan_EE469S3D_R45 (1)/S3D_Plant/ThrusterValues/FailModes/Ufail6/FailLogic ==
  BeforeFail : Inport
  FuelRemaining : Inport  Port=2
  FailMode : Inport  Port=3
  Abs : Abs  SaturateOnIntegerOverflow=off
  Compare To Constant : simulink/Logic and Bit Operations/Compare To Constant  relop=<=  const=0.5  OutDataTypeStr=boolean
  Logical Operator : Logic  Operator=OR  AllPortsSameDT=off  OutDataTypeStr=boolean
  Logical Operator1 : Logic  AllPortsSameDT=off  OutDataTypeStr=boolean
  NoFail : Outport
  wires:
  FailMode/1 -> Abs/1
  Logical Operator1/1 -> NoFail/1
  Compare To Constant/1 -> Logical Operator/2
  BeforeFail/1 -> Logical Operator/1
  Abs/1 -> Compare To Constant/1
  Logical Operator/1 -> Logical Operator1/1
  FuelRemaining/1 -> Logical Operator1/2

== system Shanthan_Heeirthan_EE469S3D_R45 (1)/S3D_Plant/ThrusterValues/FailModes/Ufail6/MAX ==
  Action Port : ActionPort  ActionPortLabel=elseif(u1 > 0.5 & u1 < 1.5)
  Constant : Constant  Value=ULIM(Udx,2)  SampleTime=dt0
  Out1 : Outport
  wires:
  Constant/1 -> Out1/1

== system Shanthan_Heeirthan_EE469S3D_R45 (1)/S3D_Plant/ThrusterValues/FailModes/Ufail6/MIN ==
  Action Port : ActionPort  ActionPortLabel=if(u1 < -0.5)
  Constant : Constant  Value=ULIM(Udx,1)  SampleTime=dt0
  Out1 : Outport
  wires:
  Constant/1 -> Out1/1

== system Shanthan_Heeirthan_EE469S3D_R45 (1)/S3D_Plant/ThrusterValues/FailModes/Ufail7/CURRENT ==
  In1 : Inport
  Action Port : ActionPort  ActionPortLabel=else
  Out1 : Outport
  wires:
  In1/1 -> Out1/1

== system Shanthan_Heeirthan_EE469S3D_R45 (1)/S3D_Plant/ThrusterValues/FailModes/Ufail7/FailLogic ==
  BeforeFail : Inport
  FuelRemaining : Inport  Port=2
  FailMode : Inport  Port=3
  Abs : Abs  SaturateOnIntegerOverflow=off
  Compare To Constant : simulink/Logic and Bit Operations/Compare To Constant  relop=<=  const=0.5  OutDataTypeStr=boolean
  Logical Operator : Logic  Operator=OR  AllPortsSameDT=off  OutDataTypeStr=boolean
  Logical Operator1 : Logic  AllPortsSameDT=off  OutDataTypeStr=boolean
  NoFail : Outport
  wires:
  FailMode/1 -> Abs/1
  Logical Operator1/1 -> NoFail/1
  Compare To Constant/1 -> Logical Operator/2
  BeforeFail/1 -> Logical Operator/1
  Abs/1 -> Compare To Constant/1
  Logical Operator/1 -> Logical Operator1/1
  FuelRemaining/1 -> Logical Operator1/2

== system Shanthan_Heeirthan_EE469S3D_R45 (1)/S3D_Plant/ThrusterValues/FailModes/Ufail7/MAX ==
  Action Port : ActionPort  ActionPortLabel=elseif(u1 > 0.5 & u1 < 1.5)
  Constant : Constant  Value=ULIM(Udx,2)  SampleTime=dt0
  Out1 : Outport
  wires:
  Constant/1 -> Out1/1

== system Shanthan_Heeirthan_EE469S3D_R45 (1)/S3D_Plant/ThrusterValues/FailModes/Ufail7/MIN ==
  Action Port : ActionPort  ActionPortLabel=if(u1 < -0.5)
  Constant : Constant  Value=ULIM(Udx,1)  SampleTime=dt0
  Out1 : Outport
  wires:
  Constant/1 -> Out1/1

== system Shanthan_Heeirthan_EE469S3D_R45 (1)/S3D_Plant/ThrusterValues/FailModes/Ufail8/CURRENT ==
  In1 : Inport
  Action Port : ActionPort  ActionPortLabel=else
  Out1 : Outport
  wires:
  In1/1 -> Out1/1

== system Shanthan_Heeirthan_EE469S3D_R45 (1)/S3D_Plant/ThrusterValues/FailModes/Ufail8/FailLogic ==
  BeforeFail : Inport
  FuelRemaining : Inport  Port=2
  FailMode : Inport  Port=3
  Abs : Abs  SaturateOnIntegerOverflow=off
  Compare To Constant : simulink/Logic and Bit Operations/Compare To Constant  relop=<=  const=0.5  OutDataTypeStr=boolean
  Logical Operator : Logic  Operator=OR  AllPortsSameDT=off  OutDataTypeStr=boolean
  Logical Operator1 : Logic  AllPortsSameDT=off  OutDataTypeStr=boolean
  NoFail : Outport
  wires:
  FailMode/1 -> Abs/1
  Logical Operator1/1 -> NoFail/1
  Compare To Constant/1 -> Logical Operator/2
  BeforeFail/1 -> Logical Operator/1
  Abs/1 -> Compare To Constant/1
  Logical Operator/1 -> Logical Operator1/1
  FuelRemaining/1 -> Logical Operator1/2

== system Shanthan_Heeirthan_EE469S3D_R45 (1)/S3D_Plant/ThrusterValues/FailModes/Ufail8/MAX ==
  Action Port : ActionPort  ActionPortLabel=elseif(u1 > 0.5 & u1 < 1.5)
  Constant : Constant  Value=ULIM(Udx,2)  SampleTime=dt0
  Out1 : Outport
  wires:
  Constant/1 -> Out1/1

== system Shanthan_Heeirthan_EE469S3D_R45 (1)/S3D_Plant/ThrusterValues/FailModes/Ufail8/MIN ==
  Action Port : ActionPort  ActionPortLabel=if(u1 < -0.5)
  Constant : Constant  Value=ULIM(Udx,1)  SampleTime=dt0
  Out1 : Outport
  wires:
  Constant/1 -> Out1/1

== system Shanthan_Heeirthan_EE469S3D_R45 (1)/S3D_Plant/ThrusterValues/FailModes/Ufail9/CURRENT ==
  In1 : Inport
  Action Port : ActionPort  ActionPortLabel=else
  Out1 : Outport
  wires:
  In1/1 -> Out1/1

== system Shanthan_Heeirthan_EE469S3D_R45 (1)/S3D_Plant/ThrusterValues/FailModes/Ufail9/FailLogic ==
  BeforeFail : Inport
  FuelRemaining : Inport  Port=2
  FailMode : Inport  Port=3
  Abs : Abs  SaturateOnIntegerOverflow=off
  Compare To Constant : simulink/Logic and Bit Operations/Compare To Constant  relop=<=  const=0.5  OutDataTypeStr=boolean
  Logical Operator : Logic  Operator=OR  AllPortsSameDT=off  OutDataTypeStr=boolean
  Logical Operator1 : Logic  AllPortsSameDT=off  OutDataTypeStr=boolean
  NoFail : Outport
  wires:
  FailMode/1 -> Abs/1
  Logical Operator1/1 -> NoFail/1
  Compare To Constant/1 -> Logical Operator/2
  BeforeFail/1 -> Logical Operator/1
  Abs/1 -> Compare To Constant/1
  Logical Operator/1 -> Logical Operator1/1
  FuelRemaining/1 -> Logical Operator1/2

== system Shanthan_Heeirthan_EE469S3D_R45 (1)/S3D_Plant/ThrusterValues/FailModes/Ufail9/MAX ==
  Action Port : ActionPort  ActionPortLabel=elseif(u1 > 0.5 & u1 < 1.5)
  Constant : Constant  Value=ULIM(Udx,2)  SampleTime=dt0
  Out1 : Outport
  wires:
  Constant/1 -> Out1/1

== system Shanthan_Heeirthan_EE469S3D_R45 (1)/S3D_Plant/ThrusterValues/FailModes/Ufail9/MIN ==
  Action Port : ActionPort  ActionPortLabel=if(u1 < -0.5)
  Constant : Constant  Value=ULIM(Udx,1)  SampleTime=dt0
  Out1 : Outport
  wires:
  Constant/1 -> Out1/1

== system Shanthan_Heeirthan_EE469S3D_R45 (1)/S3D_Plant/ThrusterValues/HealthMonitoring/DetectFailures/Subsystem ==
  UCMD : Inport
  U : Inport  Port=2
  Abs : Abs  SaturateOnIntegerOverflow=off
  Compare To Constant : simulink/Logic and Bit Operations/Compare To Constant  relop=>=  const=HM_U  OutDataTypeStr=boolean
  Constant : Constant  Value=0
  Constant1 : Constant
  Logical Operator : Logic  Operator=OR  AllPortsSameDT=off  OutDataTypeStr=boolean
  Signal Specification : SignalSpecification  Dimensions=[1]
  Signal Specification1 : SignalSpecification  Dimensions=[1]
  Sum : Sum  Inputs=|+-
  Sum1 : Sum  Inputs=++|
  Switch : Switch  Criteria=u2 > Threshold  Threshold=.4  SaturateOnIntegerOverflow=off  InputSameDT=off
  Unit Delay1 : UnitDelay  SampleTime=dt0  HasFrameUpgradeWarning=on
  Unit Delay2 : UnitDelay  SampleTime=dt0  HasFrameUpgradeWarning=on
  Out1 : Outport
  wires:
  Abs/1 -> Switch/2
  Signal Specification1/1 -> Sum/2
  Signal Specification/1 -> Sum/1
  Constant/1 -> Switch/3
  Sum1/1 -> Switch/1
  Unit Delay1/1 -> Sum1/1
  Constant1/1 -> Sum1/2
  U/1 -> Signal Specification1/1
  Logical Operator/1 -> Unit Delay2/1, Out1/1
  Compare To Constant/1 -> Logical Operator/1
  Switch/1 -> Unit Delay1/1, Compare To Constant/1
  UCMD/1 -> Signal Specification/1
  Unit Delay2/1 -> Logical Operator/2
  Sum/1 -> Abs/1

== system Shanthan_Heeirthan_EE469S3D_R45 (1)/S3D_Plant/ThrusterValues/HealthMonitoring/DetectFailures/Subsystem1 ==
  UCMD : Inport
  U : Inport  Port=2
  Abs : Abs  SaturateOnIntegerOverflow=off
  Compare To Constant : simulink/Logic and Bit Operations/Compare To Constant  relop=>=  const=HM_U  OutDataTypeStr=boolean
  Constant : Constant  Value=0
  Constant1 : Constant
  Logical Operator : Logic  Operator=OR  AllPortsSameDT=off  OutDataTypeStr=boolean
  Signal Specification : SignalSpecification  Dimensions=[1]
  Signal Specification1 : SignalSpecification  Dimensions=[1]
  Sum : Sum  Inputs=|+-
  Sum1 : Sum  Inputs=++|
  Switch : Switch  Criteria=u2 > Threshold  Threshold=.4  SaturateOnIntegerOverflow=off  InputSameDT=off
  Unit Delay1 : UnitDelay  SampleTime=dt0  HasFrameUpgradeWarning=on
  Unit Delay2 : UnitDelay  SampleTime=dt0  HasFrameUpgradeWarning=on
  Out1 : Outport
  wires:
  Abs/1 -> Switch/2
  Signal Specification1/1 -> Sum/2
  Signal Specification/1 -> Sum/1
  Constant/1 -> Switch/3
  Sum1/1 -> Switch/1
  Unit Delay1/1 -> Sum1/1
  Constant1/1 -> Sum1/2
  U/1 -> Signal Specification1/1
  Logical Operator/1 -> Unit Delay2/1, Out1/1
  Compare To Constant/1 -> Logical Operator/1
  Switch/1 -> Unit Delay1/1, Compare To Constant/1
  UCMD/1 -> Signal Specification/1
  Unit Delay2/1 -> Logical Operator/2
  Sum/1 -> Abs/1

== system Shanthan_Heeirthan_EE469S3D_R45 (1)/S3D_Plant/ThrusterValues/HealthMonitoring/DetectFailures/Subsystem2 ==
  UCMD : Inport
  U : Inport  Port=2
  Abs : Abs  SaturateOnIntegerOverflow=off
  Compare To Constant : simulink/Logic and Bit Operations/Compare To Constant  relop=>=  const=HM_U  OutDataTypeStr=boolean
  Constant : Constant  Value=0
  Constant1 : Constant
  Logical Operator : Logic  Operator=OR  AllPortsSameDT=off  OutDataTypeStr=boolean
  Signal Specification : SignalSpecification  Dimensions=[1]
  Signal Specification1 : SignalSpecification  Dimensions=[1]
  Sum : Sum  Inputs=|+-
  Sum1 : Sum  Inputs=++|
  Switch : Switch  Criteria=u2 > Threshold  Threshold=.4  SaturateOnIntegerOverflow=off  InputSameDT=off
  Unit Delay1 : UnitDelay  SampleTime=dt0  HasFrameUpgradeWarning=on
  Unit Delay2 : UnitDelay  SampleTime=dt0  HasFrameUpgradeWarning=on
  Out1 : Outport
  wires:
  Abs/1 -> Switch/2
  Signal Specification1/1 -> Sum/2
  Signal Specification/1 -> Sum/1
  Constant/1 -> Switch/3
  Sum1/1 -> Switch/1
  Unit Delay1/1 -> Sum1/1
  Constant1/1 -> Sum1/2
  U/1 -> Signal Specification1/1
  Logical Operator/1 -> Unit Delay2/1, Out1/1
  Compare To Constant/1 -> Logical Operator/1
  Switch/1 -> Unit Delay1/1, Compare To Constant/1
  UCMD/1 -> Signal Specification/1
  Unit Delay2/1 -> Logical Operator/2
  Sum/1 -> Abs/1

== system Shanthan_Heeirthan_EE469S3D_R45 (1)/S3D_Plant/ThrusterValues/HealthMonitoring/DetectFailures/Subsystem3 ==
  UCMD : Inport
  U : Inport  Port=2
  Abs : Abs  SaturateOnIntegerOverflow=off
  Compare To Constant : simulink/Logic and Bit Operations/Compare To Constant  relop=>=  const=HM_U  OutDataTypeStr=boolean
  Constant : Constant  Value=0
  Constant1 : Constant
  Logical Operator : Logic  Operator=OR  AllPortsSameDT=off  OutDataTypeStr=boolean
  Signal Specification : SignalSpecification  Dimensions=[1]
  Signal Specification1 : SignalSpecification  Dimensions=[1]
  Sum : Sum  Inputs=|+-
  Sum1 : Sum  Inputs=++|
  Switch : Switch  Criteria=u2 > Threshold  Threshold=.4  SaturateOnIntegerOverflow=off  InputSameDT=off
  Unit Delay1 : UnitDelay  SampleTime=dt0  HasFrameUpgradeWarning=on
  Unit Delay2 : UnitDelay  SampleTime=dt0  HasFrameUpgradeWarning=on
  Out1 : Outport
  wires:
  Abs/1 -> Switch/2
  Signal Specification1/1 -> Sum/2
  Signal Specification/1 -> Sum/1
  Constant/1 -> Switch/3
  Sum1/1 -> Switch/1
  Unit Delay1/1 -> Sum1/1
  Constant1/1 -> Sum1/2
  U/1 -> Signal Specification1/1
  Logical Operator/1 -> Unit Delay2/1, Out1/1
  Compare To Constant/1 -> Logical Operator/1
  Switch/1 -> Unit Delay1/1, Compare To Constant/1
  UCMD/1 -> Signal Specification/1
  Unit Delay2/1 -> Logical Operator/2
  Sum/1 -> Abs/1

== system Shanthan_Heeirthan_EE469S3D_R45 (1)/S3D_Plant/ThrusterValues/HealthMonitoring/DetectFailures/Subsystem4 ==
  UCMD : Inport
  U : Inport  Port=2
  Abs : Abs  SaturateOnIntegerOverflow=off
  Compare To Constant : simulink/Logic and Bit Operations/Compare To Constant  relop=>=  const=HM_U  OutDataTypeStr=boolean
  Constant : Constant  Value=0
  Constant1 : Constant
  Logical Operator : Logic  Operator=OR  AllPortsSameDT=off  OutDataTypeStr=boolean
  Signal Specification : SignalSpecification  Dimensions=[1]
  Signal Specification1 : SignalSpecification  Dimensions=[1]
  Sum : Sum  Inputs=|+-
  Sum1 : Sum  Inputs=++|
  Switch : Switch  Criteria=u2 > Threshold  Threshold=.4  SaturateOnIntegerOverflow=off  InputSameDT=off
  Unit Delay1 : UnitDelay  SampleTime=dt0  HasFrameUpgradeWarning=on
  Unit Delay2 : UnitDelay  SampleTime=dt0  HasFrameUpgradeWarning=on
  Out1 : Outport
  wires:
  Abs/1 -> Switch/2
  Signal Specification1/1 -> Sum/2
  Signal Specification/1 -> Sum/1
  Constant/1 -> Switch/3
  Sum1/1 -> Switch/1
  Unit Delay1/1 -> Sum1/1
  Constant1/1 -> Sum1/2
  U/1 -> Signal Specification1/1
  Logical Operator/1 -> Unit Delay2/1, Out1/1
  Compare To Constant/1 -> Logical Operator/1
  Switch/1 -> Unit Delay1/1, Compare To Constant/1
  UCMD/1 -> Signal Specification/1
  Unit Delay2/1 -> Logical Operator/2
  Sum/1 -> Abs/1

== system Shanthan_Heeirthan_EE469S3D_R45 (1)/S3D_Plant/ThrusterValues/HealthMonitoring/DetectFailures/Subsystem5 ==
  UCMD : Inport
  U : Inport  Port=2
  Abs : Abs  SaturateOnIntegerOverflow=off
  Compare To Constant : simulink/Logic and Bit Operations/Compare To Constant  relop=>=  const=HM_U  OutDataTypeStr=boolean
  Constant : Constant  Value=0
  Constant1 : Constant
  Logical Operator : Logic  Operator=OR  AllPortsSameDT=off  OutDataTypeStr=boolean
  Signal Specification : SignalSpecification  Dimensions=[1]
  Signal Specification1 : SignalSpecification  Dimensions=[1]
  Sum : Sum  Inputs=|+-
  Sum1 : Sum  Inputs=++|
  Switch : Switch  Criteria=u2 > Threshold  Threshold=.4  SaturateOnIntegerOverflow=off  InputSameDT=off
  Unit Delay1 : UnitDelay  SampleTime=dt0  HasFrameUpgradeWarning=on
  Unit Delay2 : UnitDelay  SampleTime=dt0  HasFrameUpgradeWarning=on
  Out1 : Outport
  wires:
  Abs/1 -> Switch/2
  Signal Specification1/1 -> Sum/2
  Signal Specification/1 -> Sum/1
  Constant/1 -> Switch/3
  Sum1/1 -> Switch/1
  Unit Delay1/1 -> Sum1/1
  Constant1/1 -> Sum1/2
  U/1 -> Signal Specification1/1
  Logical Operator/1 -> Unit Delay2/1, Out1/1
  Compare To Constant/1 -> Logical Operator/1
  Switch/1 -> Unit Delay1/1, Compare To Constant/1
  UCMD/1 -> Signal Specification/1
  Unit Delay2/1 -> Logical Operator/2
  Sum/1 -> Abs/1

== system Shanthan_Heeirthan_EE469S3D_R45 (1)/S3D_Plant/ThrusterValues/HealthMonitoring/DetectFailures/Subsystem6 ==
  UCMD : Inport
  U : Inport  Port=2
  Abs : Abs  SaturateOnIntegerOverflow=off
  Compare To Constant : simulink/Logic and Bit Operations/Compare To Constant  relop=>=  const=HM_U  OutDataTypeStr=boolean
  Constant : Constant  Value=0
  Constant1 : Constant
  Logical Operator : Logic  Operator=OR  AllPortsSameDT=off  OutDataTypeStr=boolean
  Signal Specification : SignalSpecification  Dimensions=[1]
  Signal Specification1 : SignalSpecification  Dimensions=[1]
  Sum : Sum  Inputs=|+-
  Sum1 : Sum  Inputs=++|
  Switch : Switch  Criteria=u2 > Threshold  Threshold=.4  SaturateOnIntegerOverflow=off  InputSameDT=off
  Unit Delay1 : UnitDelay  SampleTime=dt0  HasFrameUpgradeWarning=on
  Unit Delay2 : UnitDelay  SampleTime=dt0  HasFrameUpgradeWarning=on
  Out1 : Outport
  wires:
  Abs/1 -> Switch/2
  Signal Specification1/1 -> Sum/2
  Signal Specification/1 -> Sum/1
  Constant/1 -> Switch/3
  Sum1/1 -> Switch/1
  Unit Delay1/1 -> Sum1/1
  Constant1/1 -> Sum1/2
  U/1 -> Signal Specification1/1
  Logical Operator/1 -> Unit Delay2/1, Out1/1
  Compare To Constant/1 -> Logical Operator/1
  Switch/1 -> Unit Delay1/1, Compare To Constant/1
  UCMD/1 -> Signal Specification/1
  Unit Delay2/1 -> Logical Operator/2
  Sum/1 -> Abs/1

== system Shanthan_Heeirthan_EE469S3D_R45 (1)/S3D_Plant/ThrusterValues/HealthMonitoring/DetectFailures/Subsystem7 ==
  UCMD : Inport
  U : Inport  Port=2
  Abs : Abs  SaturateOnIntegerOverflow=off
  Compare To Constant : simulink/Logic and Bit Operations/Compare To Constant  relop=>=  const=HM_U  OutDataTypeStr=boolean
  Constant : Constant  Value=0
  Constant1 : Constant
  Logical Operator : Logic  Operator=OR  AllPortsSameDT=off  OutDataTypeStr=boolean
  Signal Specification : SignalSpecification  Dimensions=[1]
  Signal Specification1 : SignalSpecification  Dimensions=[1]
  Sum : Sum  Inputs=|+-
  Sum1 : Sum  Inputs=++|
  Switch : Switch  Criteria=u2 > Threshold  Threshold=.4  SaturateOnIntegerOverflow=off  InputSameDT=off
  Unit Delay1 : UnitDelay  SampleTime=dt0  HasFrameUpgradeWarning=on
  Unit Delay2 : UnitDelay  SampleTime=dt0  HasFrameUpgradeWarning=on
  Out1 : Outport
  wires:
  Abs/1 -> Switch/2
  Signal Specification1/1 -> Sum/2
  Signal Specification/1 -> Sum/1
  Constant/1 -> Switch/3
  Sum1/1 -> Switch/1
  Unit Delay1/1 -> Sum1/1
  Constant1/1 -> Sum1/2
  U/1 -> Signal Specification1/1
  Logical Operator/1 -> Unit Delay2/1, Out1/1
  Compare To Constant/1 -> Logical Operator/1
  Switch/1 -> Unit Delay1/1, Compare To Constant/1
  UCMD/1 -> Signal Specification/1
  Unit Delay2/1 -> Logical Operator/2
  Sum/1 -> Abs/1

== system Shanthan_Heeirthan_EE469S3D_R45 (1)/S3D_Plant/ThrusterValues/HealthMonitoring/DetectFailures/Subsystem8 ==
  UCMD : Inport
  U : Inport  Port=2
  Abs : Abs  SaturateOnIntegerOverflow=off
  Compare To Constant : simulink/Logic and Bit Operations/Compare To Constant  relop=>=  const=HM_U  OutDataTypeStr=boolean
  Constant : Constant  Value=0
  Constant1 : Constant
  Logical Operator : Logic  Operator=OR  AllPortsSameDT=off  OutDataTypeStr=boolean
  Signal Specification : SignalSpecification  Dimensions=[1]
  Signal Specification1 : SignalSpecification  Dimensions=[1]
  Sum : Sum  Inputs=|+-
  Sum1 : Sum  Inputs=++|
  Switch : Switch  Criteria=u2 > Threshold  Threshold=.4  SaturateOnIntegerOverflow=off  InputSameDT=off
  Unit Delay1 : UnitDelay  SampleTime=dt0  HasFrameUpgradeWarning=on
  Unit Delay2 : UnitDelay  SampleTime=dt0  HasFrameUpgradeWarning=on
  Out1 : Outport
  wires:
  Abs/1 -> Switch/2
  Signal Specification1/1 -> Sum/2
  Signal Specification/1 -> Sum/1
  Constant/1 -> Switch/3
  Sum1/1 -> Switch/1
  Unit Delay1/1 -> Sum1/1
  Constant1/1 -> Sum1/2
  U/1 -> Signal Specification1/1
  Logical Operator/1 -> Unit Delay2/1, Out1/1
  Compare To Constant/1 -> Logical Operator/1
  Switch/1 -> Unit Delay1/1, Compare To Constant/1
  UCMD/1 -> Signal Specification/1
  Unit Delay2/1 -> Logical Operator/2
  Sum/1 -> Abs/1

== system Shanthan_Heeirthan_EE469S3D_R45 (1)/S3D_Plant/ThrusterValues/HealthMonitoring/DetectFailures/Subsystem9 ==
  UCMD : Inport
  U : Inport  Port=2
  Abs : Abs  SaturateOnIntegerOverflow=off
  Compare To Constant : simulink/Logic and Bit Operations/Compare To Constant  relop=>=  const=HM_U  OutDataTypeStr=boolean
  Constant : Constant  Value=0
  Constant1 : Constant
  Logical Operator : Logic  Operator=OR  AllPortsSameDT=off  OutDataTypeStr=boolean
  Signal Specification : SignalSpecification  Dimensions=[1]
  Signal Specification1 : SignalSpecification  Dimensions=[1]
  Sum : Sum  Inputs=|+-
  Sum1 : Sum  Inputs=++|
  Switch : Switch  Criteria=u2 > Threshold  Threshold=.4  SaturateOnIntegerOverflow=off  InputSameDT=off
  Unit Delay1 : UnitDelay  SampleTime=dt0  HasFrameUpgradeWarning=on
  Unit Delay2 : UnitDelay  SampleTime=dt0  HasFrameUpgradeWarning=on
  Out1 : Outport
  wires:
  Abs/1 -> Switch/2
  Signal Specification1/1 -> Sum/2
  Signal Specification/1 -> Sum/1
  Constant/1 -> Switch/3
  Sum1/1 -> Switch/1
  Unit Delay1/1 -> Sum1/1
  Constant1/1 -> Sum1/2
  U/1 -> Signal Specification1/1
  Logical Operator/1 -> Unit Delay2/1, Out1/1
  Compare To Constant/1 -> Logical Operator/1
  Switch/1 -> Unit Delay1/1, Compare To Constant/1
  UCMD/1 -> Signal Specification/1
  Unit Delay2/1 -> Logical Operator/2
  Sum/1 -> Abs/1

== system Shanthan_Heeirthan_EE469S3D_R45 (1)/control_law/CMD/CMDprocess/CommandTypes/Enabled Subsystem ==
  Pdata : Inport
  Enable : EnablePort
  Bus Creator : BusCreator  Inputs=3
  Demux : Demux  Outputs=3
  ICs : Outport
  wires:
  Pdata/1 -> Demux/1
  Demux/1 -> Bus Creator/1  "ICX"
  Demux/2 -> Bus Creator/2  "ICY"
  Demux/3 -> Bus Creator/3  "ICZ"
  Bus Creator/1 -> ICs/1  "ICs"
